simulink model "Mars_sim"  (R2024b)
settings: Solver=VariableStepAuto  StartTime=0.0  StopTime=5e5  MaxStep=50  RelTol=1e-6
values from neighbouring files (symbols this model uses):
  capture = delta_v*rot*v_orbiter/norm(v_orbiter)    [Mars_setup.m]
  Mars_planet = Planet(mu,R,s,0,0)    [Mars_capture_setup.m]    (also in Mars_setup.m)
settings Model: Creator=cpero  LastModifiedBy=cpero

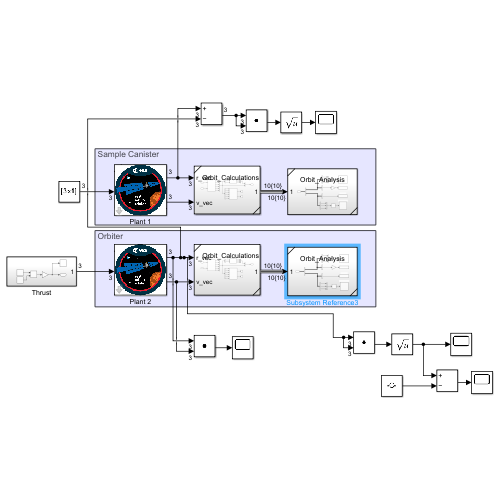
[thumbnail: Simulink's stored preview of the top-level diagram]
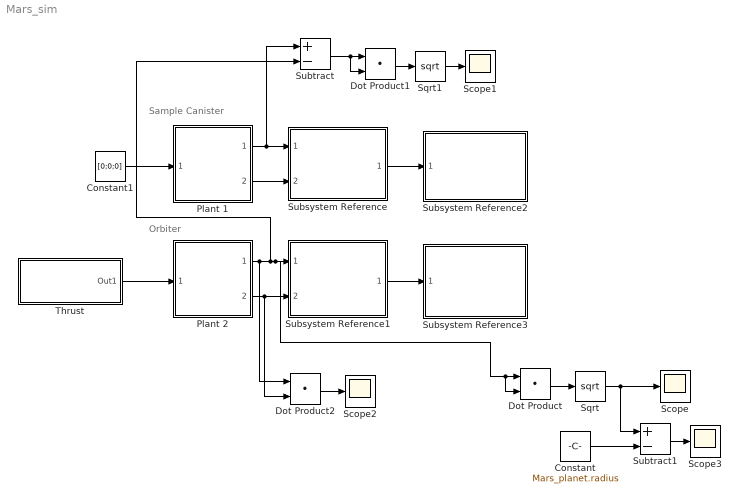
== system Mars_sim ==
  note: Orbiter
  note: Sample Canister
  Constant : Constant  Value=Mars_planet.radius
  Constant1 : Constant  Value=[0;0;0]
  Dot Product : DotProduct  OutDataTypeStr=Inherit: Inherit via internal rule
  Dot Product1 : DotProduct  OutDataTypeStr=Inherit: Inherit via internal rule
  Dot Product2 : DotProduct  OutDataTypeStr=Inherit: Inherit via internal rule
  Plant 1 : Subsystem  ReferencedSubsystem=Plant  initial_data=canister_initial  maneuver_time=0  mu=Mars_planet.mu
  Plant 2 : Subsystem  ReferencedSubsystem=Plant  initial_data=orbiter_initial  maneuver_time=0  mu=Mars_planet.mu
  Scope{,1..3} (4 alike) : Scope
  Sqrt : Sqrt
  Sqrt1 : Sqrt
  Subsystem Reference : Subsystem  ReferencedSubsystem=Orbit_Calculations
  Subsystem Reference1 : Subsystem  ReferencedSubsystem=Orbit_Calculations
  Subsystem Reference2 : Subsystem  ReferencedSubsystem=Orbit_Analysis
  Subsystem Reference3 : Subsystem  ReferencedSubsystem=Orbit_Analysis
  Subtract : Sum  Inputs=+-
  Subtract1 : Sum  Inputs=+-
  Thrust : Subsystem
  wires:
  Plant 1/1 -> Subtract/1, Subsystem Reference/1
  Plant 2/1 -> Dot Product2/1, Subsystem Reference1/1, Dot Product/2, Dot Product/1, Subtract/2
  Plant 2/2 -> Dot Product2/2, Subsystem Reference1/2
  Plant 1/2 -> Subsystem Reference/2
  Thrust/1(Out1) -> Plant 2/1
  Constant1/1 -> Plant 1/1
  Dot Product/1 -> Sqrt/1
  Sqrt/1 -> Subtract1/1, Scope/1
  Subsystem Reference/1 -> Subsystem Reference2/1
  Subsystem Reference1/1 -> Subsystem Reference3/1
  Subtract/1 -> Dot Product1/2, Dot Product1/1
  Dot Product1/1 -> Sqrt1/1
  Sqrt1/1 -> Scope1/1
  Dot Product2/1 -> Scope2/1
  Constant/1 -> Subtract1/2
  Subtract1/1 -> Scope3/1

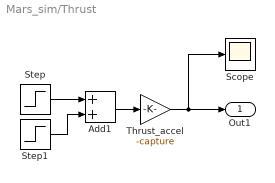
== system Mars_sim/Thrust ==
  Add1 : Sum
  Scope : Scope
  Step : Step  Time=3.714e5  SampleTime=0
  Step1 : Step  Time=3.714e5 + 1  After=-1  SampleTime=0
  Thrust_accel : Gain  Gain=-capture
  Out1 : Outport
  wires:
  Add1/1 -> Thrust_accel/1
  Thrust_accel/1 -> Out1/1, Scope/1
  Step1/1 -> Add1/2
  Step/1 -> Add1/1
